simulink model "modelo"  (Simulink 7.7)
settings: Solver=ode45  StartTime=0.0  StopTime=40  MaxStep=1e-3  RelTol=1e-3
values from neighbouring files (symbols this model uses):
  Kenc = 3.18309886184    [matlab.mat]    (also in resumo.m)
  Km = 3.12779302234    [matlab.mat]    (also in resumo.m)
  Ktac = 0.255103132162    [matlab.mat]    (also in resumo.m)
  taum = 0.43    [matlab.mat]    (also in resumo.m)
settings Model: Creator=03135  LastModifiedBy=03135

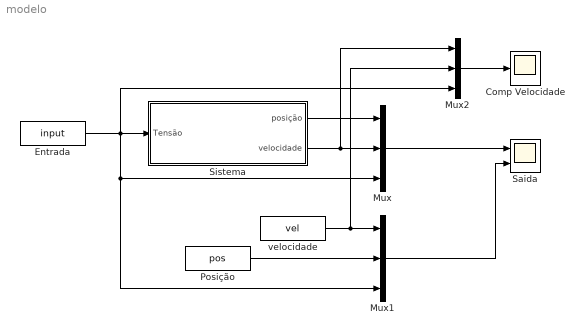
== system modelo ==
  Comp Velocidade : Scope
  Entrada : FromWorkspace  VariableName=input  SampleTime=0
  Mux : Mux  Inputs=3
  Mux1 : Mux  Inputs=3
  Mux2 : Mux  Inputs=3
  Posição : FromWorkspace  VariableName=pos  SampleTime=0
  Saida : Scope  NumInputPorts=2
      settings: YMin=-5~-5  YMax=5~5
  Sistema : Subsystem
  velocidade : FromWorkspace  VariableName=vel  SampleTime=0
  wires:
  Mux/1 -> Saida/1
  Sistema/1(posição) -> Mux/1
  Sistema/2(velocidade) -> Mux/2, Mux2/1
  Entrada/1 -> Sistema/1(Tensão), Mux/3, Mux1/3, Mux2/3
  Mux1/1 -> Saida/2
  velocidade/1 -> Mux1/1, Mux2/2
  Posição/1 -> Mux1/2
  Mux2/1 -> Comp Velocidade/1

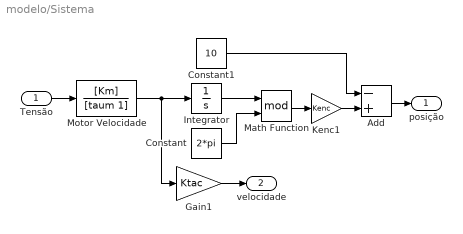
== system modelo/Sistema ==
  Tensão : Inport
  Add : Sum  Inputs=-+
  Constant : Constant  Value=2*pi
  Constant1 : Constant  Value=10
  Gain1 : Gain  Gain=Ktac
  Integrator : Integrator
  Kenc1 : Gain  Gain=Kenc
  Math Function : Math  Operator=mod  SaturateOnIntegerOverflow=on
  Motor Velocidade : TransferFcn  Numerator=[Km]  Denominator=[taum 1]
  posição : Outport
  velocidade : Outport  Port=2
  wires:
  Motor Velocidade/1 -> Integrator/1, Gain1/1
  Tensão/1 -> Motor Velocidade/1
  Gain1/1 -> velocidade/1
  Math Function/1 -> Kenc1/1
  Integrator/1 -> Math Function/1
  Constant/1 -> Math Function/2
  Add/1 -> posição/1
  Kenc1/1 -> Add/2
  Constant1/1 -> Add/1
